simulink model "Buck_COMPEL_2019"  (R2019b)
settings: Solver=VariableStepAuto  StartTime=0.0  StopTime=Ts  RelTol=1e-3
undefined symbols (not defined in the file or in its folder): fixed, plecs
libraries: plecslib_extras2 x1
settings Model: Creator=jbaxte24  LastModifiedBy=jb
settings DataIOCC: ReturnWorkspaceOutputs=off
settings DebuggingCC: ArithmeticOperatorsInVariantConditions=warning
settings SFSimCC: SimUseLocalCustomCode=off  CustomCodeUndefinedFunction=UseInterfaceOnly
settings RTWCC: RTWUseLocalCustomCode=off
settings CodeAppCC: StateflowObjectComments=on

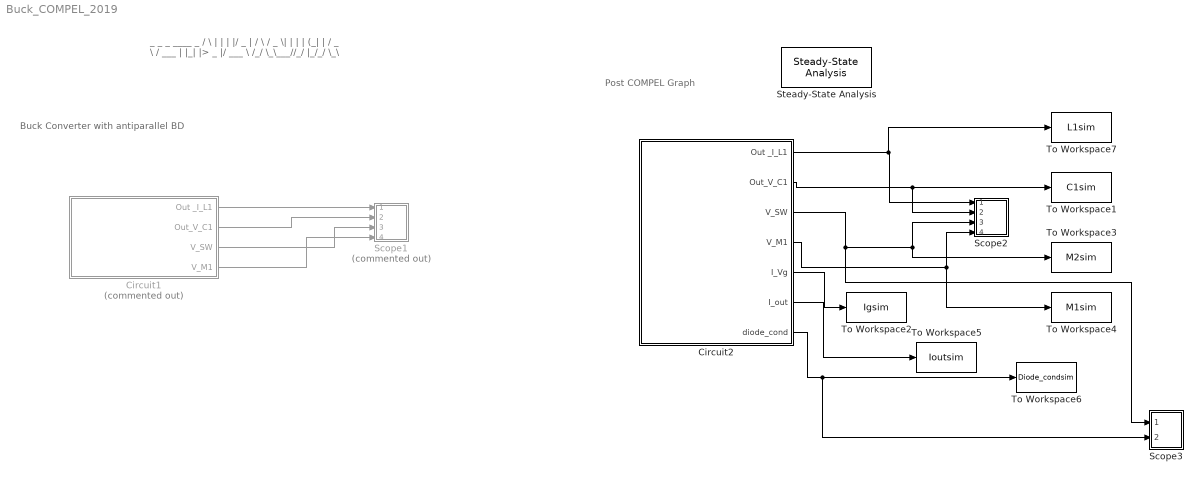
== system Buck_COMPEL_2019 ==
  note: Post COMPEL Graph
  note: Buck Converter with antiparallel BD
  note: _ _ _ ____ _
      | / \ | | | |/ _ | / \
      | / _ \| | | | (_| | / _ \
      | / ___ | |_| |> _ |/ ___ \
      | /_/ \_\___//_/ |_/_/ \_\
  Circuit1 : Subsystem  Commented=on  LoadFcn=plecs('sl', 200);  InitFcn=plecs('sl', 214);  StartFcn=plecs('sl', 208);  StopFcn=plecs('sl', 209);  mask(PlecsCircuit){PLECSData=<binary blob, 2572 chars, not shown>}
      mask prompts: PLECSData "PLECS Data (Do not delete or modify!)"
      mask init:
      | % PLACE CUSTOM INITIALIZATIONS ABOVE
      | % DO NOT REMOVE
      | plecs('sl', 215);
      | % DO NOT REMOVE
      settings: CopyFcn=plecs('sl', 203);  DeleteFcn=plecs('sl', 205);  UndoDeleteFcn=plecs('sl', 206);  PreSaveFcn=plecs('sl', 211);  PostSaveFcn=plecs('sl', 201);  NameChangeFcn=plecs('sl', 210);  DestroyFcn=plecs('sl', 207);  PreCopyFcn=plecs('sl', 216);  OpenFcn=plecs('sl', 202);  ErrorFcn=plerrorfcn
      mask Help: web(['file:///' fullfile(plecsdoc, 'creatingacircuit.html')])
      mask Display: disp('PLECS\nCircuit')
  Circuit2 : Subsystem  LoadFcn=plecs('sl', 200);  InitFcn=plecs('sl', 214);  StartFcn=plecs('sl', 208);  StopFcn=plecs('sl', 209);  mask(PlecsCircuit){PLECSData=<binary blob, 2928 chars, not shown>}
      mask prompts: PLECSData "PLECS Data (Do not delete or modify!)"
      mask init:
      | % PLACE CUSTOM INITIALIZATIONS ABOVE
      | % DO NOT REMOVE
      | plecs('sl', 215);
      | % DO NOT REMOVE
      settings: CopyFcn=plecs('sl', 203);  DeleteFcn=plecs('sl', 205);  UndoDeleteFcn=plecs('sl', 206);  PreSaveFcn=plecs('sl', 211);  PostSaveFcn=plecs('sl', 201);  NameChangeFcn=plecs('sl', 210);  DestroyFcn=plecs('sl', 207);  PreCopyFcn=plecs('sl', 216);  OpenFcn=plecs('sl', 202);  ErrorFcn=plerrorfcn
      mask Help: web(['file:///' fullfile(plecsdoc, 'creatingacircuit.html')])
      mask Display: disp('PLECS\nCircuit')
  Scope1 : Subsystem  Commented=on  LoadFcn=plecs('sl', 300);  InitFcn=plecs('sl', 314);  StartFcn=plecs('sl', 308);  StopFcn=plecs('sl', 309);  mask{Settings=<binary blob, 1468 chars, not shown>}
      mask init:
      | plecs('sl', 315);
      settings: CopyFcn=plecs('sl', 303);  DeleteFcn=plecs('sl', 305);  UndoDeleteFcn=plecs('sl', 306);  PreSaveFcn=plecs('sl', 311);  NameChangeFcn=plecs('sl', 310);  DestroyFcn=plecs('sl', 307);  OpenFcn=plecs('sl', 302);  ErrorFcn=plerrorfcn
      mask Display: plot([0.1 0.9 0.9 0.1 0.1], [0.9 0.9 0.5 0.5 0.9])
  Scope2 : Subsystem  LoadFcn=plecs('sl', 300);  InitFcn=plecs('sl', 314);  StartFcn=plecs('sl', 308);  StopFcn=plecs('sl', 309);  mask{Settings=<binary blob, 1468 chars, not shown>}
      mask init:
      | plecs('sl', 315);
      settings: CopyFcn=plecs('sl', 303);  DeleteFcn=plecs('sl', 305);  UndoDeleteFcn=plecs('sl', 306);  PreSaveFcn=plecs('sl', 311);  NameChangeFcn=plecs('sl', 310);  DestroyFcn=plecs('sl', 307);  OpenFcn=plecs('sl', 302);  ErrorFcn=plerrorfcn
      mask Display: plot([0.1 0.9 0.9 0.1 0.1], [0.9 0.9 0.5 0.5 0.9])
  Scope3 : Subsystem  LoadFcn=plecs('sl', 300);  InitFcn=plecs('sl', 314);  StartFcn=plecs('sl', 308);  StopFcn=plecs('sl', 309);  mask{Settings=<binary blob, 1188 chars, not shown>}
      mask init:
      | plecs('sl', 315);
      settings: CopyFcn=plecs('sl', 303);  DeleteFcn=plecs('sl', 305);  UndoDeleteFcn=plecs('sl', 306);  PreSaveFcn=plecs('sl', 311);  NameChangeFcn=plecs('sl', 310);  DestroyFcn=plecs('sl', 307);  OpenFcn=plecs('sl', 302);  ErrorFcn=plerrorfcn
      mask Display: plot([0.1 0.9 0.9 0.1 0.1], [0.9 0.9 0.5 0.5 0.9])
  Steady-State Analysis : plecslib_extras2/Analysis Tools/Steady-State Analysis  Period=fixed  TriggerType=rising  TimeSpan=5e-06  TStart=0  MaxIter=10000  Tolerance=1e-5  Display=off  HideScopes=off  HiddenStates=error  FinalStateName=xSteadyState  NCycles=3  JPert=1e-4  JacobianCalculation=fast  NInitCycles=0
      settings: SourceProductName=PLECS Extras
  To Workspace1 : ToWorkspace  VariableName=C1sim  SaveFormat=Timeseries  SampleTime=-1
  To Workspace2 : ToWorkspace  VariableName=Igsim  SaveFormat=Timeseries  SampleTime=-1
  To Workspace3 : ToWorkspace  VariableName=M2sim  SaveFormat=Timeseries  SampleTime=-1
  To Workspace4 : ToWorkspace  VariableName=M1sim  SaveFormat=Timeseries  SampleTime=-1
  To Workspace5 : ToWorkspace  VariableName=Ioutsim  SaveFormat=Timeseries  SampleTime=-1
  To Workspace6 : ToWorkspace  VariableName=Diode_condsim  SaveFormat=Timeseries  SampleTime=-1
  To Workspace7 : ToWorkspace  VariableName=L1sim  SaveFormat=Timeseries  SampleTime=-1
  wires:
  Circuit1/1(Out _I_L1) -> Scope1/1(1)
  Circuit1/2(Out_V_C1) -> Scope1/2(2)
  Circuit1/3(V_SW) -> Scope1/3(3)
  Circuit1/4(V_M1) -> Scope1/4(4)
  Circuit2/2(Out_V_C1) -> Scope2/2(2), To Workspace1/1
  Circuit2/4(V_M1) -> To Workspace4/1, Scope2/4(4)
  Circuit2/3(V_SW) -> Scope2/3(3), To Workspace3/1, Scope3/1(1)
  Circuit2/1(Out _I_L1) -> To Workspace7/1, Scope2/1(1)
  Circuit2/5(I_Vg) -> To Workspace2/1
  Circuit2/6(I_out) -> To Workspace5/1
  Circuit2/7(diode_cond) -> Scope3/2(2), To Workspace6/1

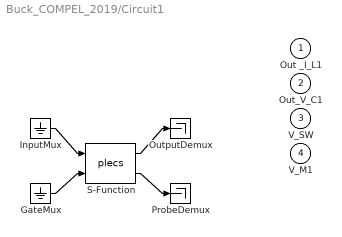
== system Buck_COMPEL_2019/Circuit1 ==
  " GateMux " : Ground
  " InputMux " : Ground
  " OutputDemux " : Terminator
  " ProbeDemux " : Terminator
  " S-Function " : S-Function  FunctionName=plecs  SFunctionDeploymentMode=off  EnableBusSupport=off
  Out _I_L1 : Outport  PortDimensions=1
  Out_V_C1 : Outport  Port=2  PortDimensions=1
  V_SW : Outport  Port=3  PortDimensions=1
  V_M1 : Outport  Port=4  PortDimensions=1
  wires:
  " InputMux "/1 -> " S-Function "/1
  " GateMux "/1 -> " S-Function "/2
  " S-Function "/1 -> " OutputDemux "/1
  " S-Function "/2 -> " ProbeDemux "/1

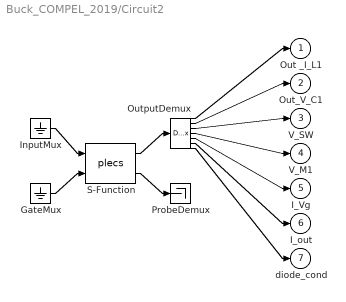
== system Buck_COMPEL_2019/Circuit2 ==
  " GateMux " : Ground
  " InputMux " : Ground
  " OutputDemux " : Demux  Outputs=[ 1 1 1 1 1 1 2 ]
  " ProbeDemux " : Terminator
  " S-Function " : S-Function  FunctionName=plecs  SFunctionDeploymentMode=off  EnableBusSupport=off
  Out _I_L1 : Outport  PortDimensions=1
  Out_V_C1 : Outport  Port=2  PortDimensions=1
  V_SW : Outport  Port=3  PortDimensions=1
  V_M1 : Outport  Port=4  PortDimensions=1
  I_Vg : Outport  Port=5  PortDimensions=1
  I_out : Outport  Port=6  PortDimensions=1
  diode_cond : Outport  Port=7  PortDimensions=2
  wires:
  " InputMux "/1 -> " S-Function "/1
  " GateMux "/1 -> " S-Function "/2
  " S-Function "/1 -> " OutputDemux "/1
  " S-Function "/2 -> " ProbeDemux "/1
  " OutputDemux "/1 -> Out _I_L1/1
  " OutputDemux "/2 -> Out_V_C1/1
  " OutputDemux "/3 -> V_SW/1
  " OutputDemux "/4 -> V_M1/1
  " OutputDemux "/5 -> I_Vg/1
  " OutputDemux "/6 -> I_out/1
  " OutputDemux "/7 -> diode_cond/1

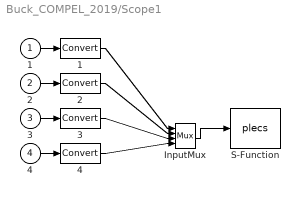
== system Buck_COMPEL_2019/Scope1 ==
  1 : Inport
  2 : Inport  Port=2
  3 : Inport  Port=3
  4 : Inport  Port=4
  " 1 " : DataTypeConversion  SaturateOnIntegerOverflow=on  RndMeth=Zero
  " 2 " : DataTypeConversion  SaturateOnIntegerOverflow=on  RndMeth=Zero
  " 3 " : DataTypeConversion  SaturateOnIntegerOverflow=on  RndMeth=Zero
  " 4 " : DataTypeConversion  SaturateOnIntegerOverflow=on  RndMeth=Zero
  " InputMux " : Mux
  " S-Function " : S-Function  FunctionName=plecs  SFunctionDeploymentMode=off  EnableBusSupport=off
  wires:
  " InputMux "/1 -> " S-Function "/1
  1/1 -> " 1 "/1
  " 1 "/1 -> " InputMux "/1
  2/1 -> " 2 "/1
  " 2 "/1 -> " InputMux "/2
  3/1 -> " 3 "/1
  " 3 "/1 -> " InputMux "/3
  4/1 -> " 4 "/1
  " 4 "/1 -> " InputMux "/4

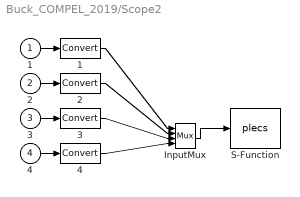
== system Buck_COMPEL_2019/Scope2 ==
  1 : Inport
  2 : Inport  Port=2
  3 : Inport  Port=3
  4 : Inport  Port=4
  " 1 " : DataTypeConversion  SaturateOnIntegerOverflow=on  RndMeth=Zero
  " 2 " : DataTypeConversion  SaturateOnIntegerOverflow=on  RndMeth=Zero
  " 3 " : DataTypeConversion  SaturateOnIntegerOverflow=on  RndMeth=Zero
  " 4 " : DataTypeConversion  SaturateOnIntegerOverflow=on  RndMeth=Zero
  " InputMux " : Mux
  " S-Function " : S-Function  FunctionName=plecs  SFunctionDeploymentMode=off  EnableBusSupport=off
  wires:
  " InputMux "/1 -> " S-Function "/1
  1/1 -> " 1 "/1
  " 1 "/1 -> " InputMux "/1
  2/1 -> " 2 "/1
  " 2 "/1 -> " InputMux "/2
  3/1 -> " 3 "/1
  " 3 "/1 -> " InputMux "/3
  4/1 -> " 4 "/1
  " 4 "/1 -> " InputMux "/4

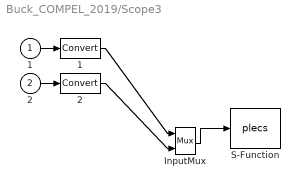
== system Buck_COMPEL_2019/Scope3 ==
  1 : Inport
  2 : Inport  Port=2
  " 1 " : DataTypeConversion  SaturateOnIntegerOverflow=on  RndMeth=Zero
  " 2 " : DataTypeConversion  SaturateOnIntegerOverflow=on  RndMeth=Zero
  " InputMux " : Mux  Inputs=2
  " S-Function " : S-Function  FunctionName=plecs  SFunctionDeploymentMode=off  EnableBusSupport=off
  wires:
  " InputMux "/1 -> " S-Function "/1
  1/1 -> " 1 "/1
  " 1 "/1 -> " InputMux "/1
  2/1 -> " 2 "/1
  " 2 "/1 -> " InputMux "/2
